simulink model "pseudonoise"  (R2014b)
settings: Solver=FixedStepDiscrete  StartTime=0.0  StopTime=0.1  FixedStep=1e-4  RelTol=1e-3
settings Model: SimulationMode=accelerator  Creator=wangsp1  LastModifiedBy=wangsp1
settings OptimizationCC: OptimizeModelRefInitCode=on  LifeSpan=Inf
settings HardwareCC: ProdIntDivRoundTo=Zero  ProdEndianess=LittleEndian  ProdHWDeviceType=Renesas->V850
settings SFSimCC: SimCustomHeaderCode=|
  | #include "syst.h"
  | #include "noisa.h"
settings SFSimCC: SimUserSources=|
  | noisa.c
  | noisa_test.c
settings RTWCC: SystemTargetFile=ert.tlc  GenCodeOnly=on  TemplateMakefile=ert_default_tmf  Description=Embedded Coder  ProcessScript=ert_make_rtw_hook  RTWUseSimCustomCode=on
settings RTWCC: CustomHeaderCode=|
  | #include "syst.h"
  | #include "noisa.h"
settings RTWCC: CustomSource=|
  | noisa.c
  | noisa_test.c
settings CodeAppCC: IgnoreCustomStorageClasses=off
settings ERTTargetCC: GenerateSampleERTMain=on  ERTCustomFileTemplate=example_file_process.tlc

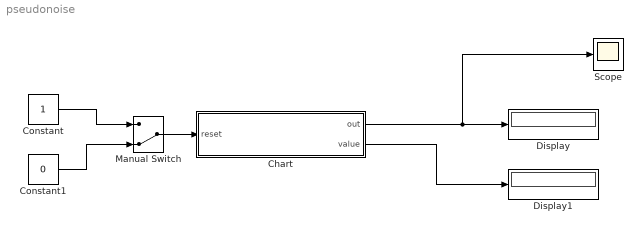
== system pseudonoise ==
  Chart : Stateflow chart  TreatAsAtomicUnit=on
  Constant : Constant  OutDataTypeStr=uint8
  Constant1 : Constant  Value=0  OutDataTypeStr=uint8
  Display : Display
  Display1 : Display
  Manual Switch : ManualSwitch  CurrentSetting=0
  Scope : Scope
      settings: YMin=0  YMax=1
  wires:
  Manual Switch/1 -> Chart/1(reset)
  Constant/1 -> Manual Switch/1
  Constant1/1 -> Manual Switch/2
  Chart/1(out) -> Scope/1, Display/1
  Chart/2(value) -> Display1/1

== stateflow chart pseudonoise/Chart ==
  (default) -> (junction 4)
  (junction 5) -> (junction 8) : {out=NOISA_Update();...
      | value=NOISA_GetValue();
      | }
  (junction 4) -> (junction 5) [order 1] : [reset==1]{NOISA_Init();}
  (junction 4) -> (junction 5) [order 2]
  data: reset input uint8; out output uint8; value output uint32
